simulink model "model"  (R2020a)
settings: Solver=ode4  StartTime=0.0  StopTime=simtime  FixedStep=0.001  RelTol=1e-3
values from neighbouring files (symbols this model uses):
  desired_energy = M1*g*(H+r1) + M2*g*(H+k0+r2)    (= 228.34)    [init.m]
  desired_energy2 = M1*g*(H2+r1) + M2*g*(H2+k0+r2)    (= 271.46)    [init.m]
  g = 9.8    [init.m]
  H = 0.8    [init.m]
  H2 = 1.2    [init.m]
  I1 = 1    [init.m]
  I2 = 10    [init.m]
  ini_theta1 = 0    [init.m]
  ini_theta1_d = 0    [init.m]
  ini_theta2 = 0    [init.m]
  ini_theta2_d = 0    [init.m]
  ini_x1 = ini_x0+r1*sin(ini_theta1)    [init.m]
  ini_x1_d = 0    [init.m]
  ini_x2 = ini_x1+r2*sin(ini_theta2)    [init.m]
  ini_x2_d = 0    [init.m]
  ini_y1 = ini_y0+r1*cos(ini_theta1)    [init.m]
  ini_y1_d = 0    [init.m]
  ini_y2 = ini_y0+ini_w+r2*cos(ini_theta2)    [init.m]
  ini_y2_d = 0    [init.m]
  M1 = 1    [init.m]
  M2 = 10    [init.m]
  r1 = 0.5    [init.m]
  r2 = 0.4    [init.m]
  T2_change = 50    [init.m]
settings Model: Creator=fabia  LastModifiedBy=Josè

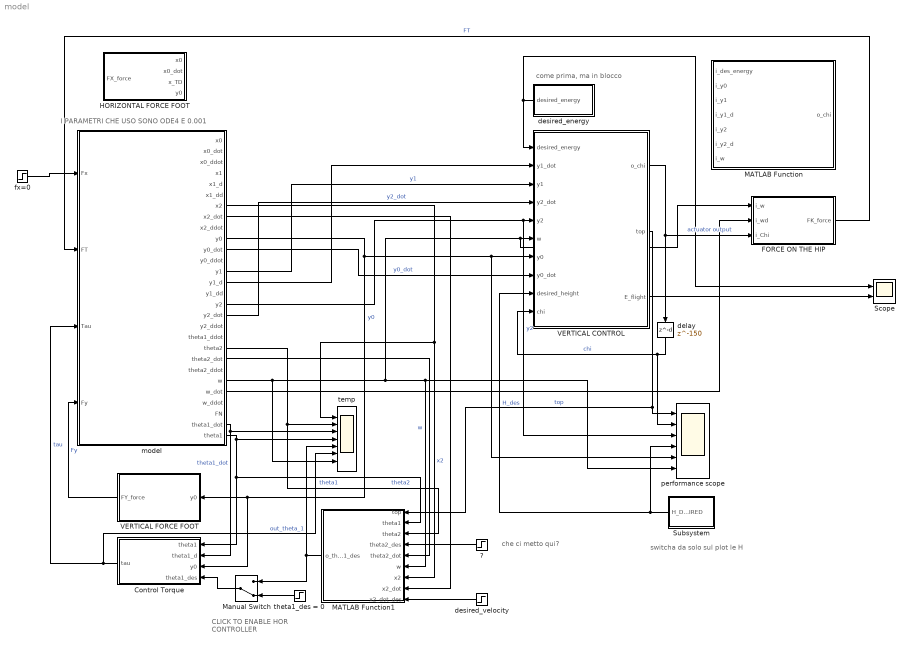
== system model ==
  note: che ci metto qui?
  note: CLICK TO ENABLE HOR CONTROLLER
  note: I PARAMETRI CHE USO SONO ODE4 E 0.001
  note: come prima, ma in blocco
  note: switcha da solo sul plot le H
  " HORIZONTAL FORCE FOOT" : MATLAB Function  TreatAsAtomicUnit=on
  " VERTICAL FORCE FOOT" : MATLAB Function  TreatAsAtomicUnit=on
  "?" : Step  Time=0  After=0  SampleTime=0
  Control Torque : MATLAB Function  TreatAsAtomicUnit=on
  FORCE ON THE HIP : MATLAB Function  TreatAsAtomicUnit=on
  MATLAB Function : MATLAB Function  TreatAsAtomicUnit=on
  MATLAB Function1 : MATLAB Function  TreatAsAtomicUnit=on
  Manual Switch : ManualSwitch  CurrentSetting=0
  Scope : Scope  NumInputPorts=2
  Subsystem : Subsystem
  VERTICAL CONTROL : MATLAB Function  TreatAsAtomicUnit=on
  delay : Delay  DelayLength=150  InitialCondition=0
  desired_energy : Subsystem
  desired_velocity : Step  Time=0  After=0.1  SampleTime=0
  fx=0 : Step  Time=0  After=0  SampleTime=0
  model : Subsystem
  performance scope : Scope  NumInputPorts=6
  temp : Scope  NumInputPorts=7
  theta1_des = 0 : Step  Time=0  After=0  SampleTime=0
  wires:
  VERTICAL CONTROL/1(o_chi) -> FORCE ON THE HIP/3(i_Chi), delay/1  "actuator output"
  fx=0/1 -> model/1(Fx)
  desired_energy/1(desired_energy) -> Scope/1, VERTICAL CONTROL/1(desired_energy)
  delay/1 -> performance scope/2, VERTICAL CONTROL/10(chi)  "chi"
  Subsystem/1(H_DESIRED) -> performance scope/4, VERTICAL CONTROL/9(desired_height)  "H_des"
  model/16(y2) -> performance scope/3, VERTICAL CONTROL/5(y2)  "y2"
  model/23(w) -> performance scope/6, MATLAB Function1/6(w), FORCE ON THE HIP/1(i_w), VERTICAL CONTROL/6(w), temp/7  "w"
  model/10(y0) -> Control Torque/3(y0), " VERTICAL FORCE FOOT"/1(y0), performance scope/5, VERTICAL CONTROL/7(y0)  "y0"
  model/11(y0_dot) -> VERTICAL CONTROL/8(y0_dot)  "y0_dot"
  model/13(y1) -> VERTICAL CONTROL/3(y1)  "y1"
  model/17(y2_dot) -> VERTICAL CONTROL/4(y2_dot)  "y2_dot"
  model/14(y1_d) -> VERTICAL CONTROL/2(y1_dot)
  " VERTICAL FORCE FOOT"/1(FY_force) -> model/4(Fy)  "Fy"
  FORCE ON THE HIP/1(FK_force) -> model/2(FT)  "FT"
  model/24(w_dot) -> FORCE ON THE HIP/2(i_wd)
  Control Torque/1(tau) -> temp/6, model/3(Tau)  "tau"
  model/28(theta1) -> MATLAB Function1/2(theta1), Control Torque/1(theta1), temp/4  "theta1"
  model/27(theta1_dot) -> Control Torque/2(theta1_d), temp/3  "theta1_dot"
  model/20(theta2) -> temp/2, MATLAB Function1/3(theta2)  "theta2"
  VERTICAL CONTROL/2(top) -> MATLAB Function1/1(top), performance scope/1  "top"
  "?"/1 -> MATLAB Function1/4(theta2_des)
  model/21(theta2_dot) -> MATLAB Function1/5(theta2_dot)
  model/7(x2) -> temp/1, MATLAB Function1/7(x2)  "x2"
  model/8(x2_dot) -> MATLAB Function1/8(x2_dot)
  desired_velocity/1 -> MATLAB Function1/9(x2_dot_des)
  MATLAB Function1/1(o_theta1_des) -> Manual Switch/1, temp/5  "out_theta_1"
  Manual Switch/1 -> Control Torque/4(theta1_des)
  theta1_des = 0/1 -> Manual Switch/2
  VERTICAL CONTROL/3(E_flight) -> Scope/2

== system model/Subsystem ==
  Add1 : Sum  Inputs=+-+
  Step1 : Step  Time=T2_change  After=H  SampleTime=0
  Step4 : Step  Time=T2_change  After=H2  SampleTime=0
  initial1 : Step  Time=0  After=H  SampleTime=0
  H_DESIRED : Outport
  wires:
  Step4/1 -> Add1/3
  Step1/1 -> Add1/2
  initial1/1 -> Add1/1
  Add1/1 -> H_DESIRED/1  "H_DESIRED"

== system model/desired_energy ==
  Add : Sum  Inputs=+-+
  Step2 : Step  Time=T2_change  After=desired_energy  SampleTime=0
  Step3 : Step  Time=T2_change  After=desired_energy2  SampleTime=0
  initial : Step  Time=0  After=desired_energy  SampleTime=0
  desired_energy : Outport
  wires:
  initial/1 -> Add/1
  Step2/1 -> Add/2
  Step3/1 -> Add/3
  Add/1 -> desired_energy/1

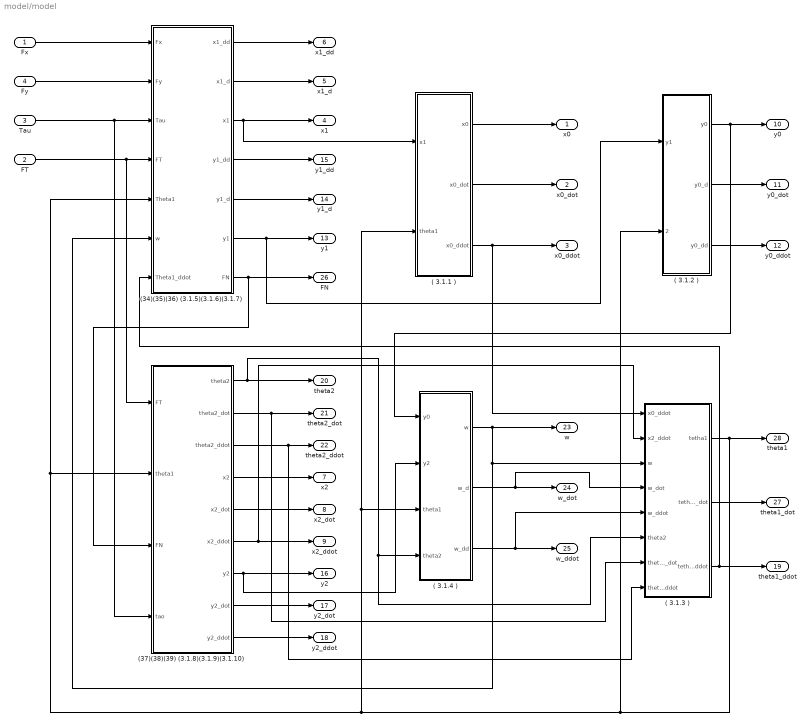
== system model/model ==
  Fx : Inport
  FT : Inport  Port=2
  Tau : Inport  Port=3
  Fy : Inport  Port=4
  "( 3.1.1 ) " : Subsystem
  ( 3.1.2 ) : Subsystem
  ( 3.1.3 ) : Subsystem
  ( 3.1.4 ) : Subsystem
  (34)(35)(36) (3.1.5)(3.1.6)(3.1.7) : Subsystem
  (37)(38)(39) (3.1.8)(3.1.9)(3.1.10) : Subsystem
  x0 : Outport
  x0_dot : Outport  Port=2
  x0_ddot : Outport  Port=3
  x1 : Outport  Port=4
  x1_d : Outport  Port=5
  x1_dd : Outport  Port=6
  x2 : Outport  Port=7
  x2_dot : Outport  Port=8
  x2_ddot : Outport  Port=9
  y0 : Outport  Port=10
  y0_dot : Outport  Port=11
  y0_ddot : Outport  Port=12
  y1 : Outport  Port=13
  y1_d : Outport  Port=14
  y1_dd : Outport  Port=15
  y2 : Outport  Port=16
  y2_dot : Outport  Port=17
  y2_ddot : Outport  Port=18
  theta1_ddot : Outport  Port=19
  theta2 : Outport  Port=20
  theta2_dot : Outport  Port=21
  theta2_ddot : Outport  Port=22
  w : Outport  Port=23
  w_dot : Outport  Port=24
  w_ddot : Outport  Port=25
  FN : Outport  Port=26
  theta1_dot : Outport  Port=27
  theta1 : Outport  Port=28
  wires:
  (34)(35)(36) (3.1.5)(3.1.6)(3.1.7)/3(x1) -> "( 3.1.1 ) "/1(x1), x1/1
  Fy/1 -> (34)(35)(36) (3.1.5)(3.1.6)(3.1.7)/2(Fy)
  Tau/1 -> (34)(35)(36) (3.1.5)(3.1.6)(3.1.7)/3(Tau), (37)(38)(39) (3.1.8)(3.1.9)(3.1.10)/4(tao)
  (34)(35)(36) (3.1.5)(3.1.6)(3.1.7)/4(y1_dd) -> y1_dd/1
  "( 3.1.1 ) "/1(x0) -> x0/1
  (34)(35)(36) (3.1.5)(3.1.6)(3.1.7)/5(y1_d) -> y1_d/1
  (34)(35)(36) (3.1.5)(3.1.6)(3.1.7)/6(y1) -> ( 3.1.2 )/1(y1), y1/1
  Fx/1 -> (34)(35)(36) (3.1.5)(3.1.6)(3.1.7)/1(Fx)
  (34)(35)(36) (3.1.5)(3.1.6)(3.1.7)/1(x1_dd) -> x1_dd/1
  "( 3.1.1 ) "/2(x0_dot) -> x0_dot/1
  (34)(35)(36) (3.1.5)(3.1.6)(3.1.7)/2(x1_d) -> x1_d/1
  (34)(35)(36) (3.1.5)(3.1.6)(3.1.7)/7(FN) -> (37)(38)(39) (3.1.8)(3.1.9)(3.1.10)/3(FN), FN/1
  "( 3.1.1 ) "/3(x0_ddot) -> x0_ddot/1, ( 3.1.3 )/1(x0_ddot)
  ( 3.1.2 )/1(y0) -> ( 3.1.4 )/1(y0), y0/1
  ( 3.1.2 )/2(y0_d) -> y0_dot/1
  ( 3.1.2 )/3(y0_dd) -> y0_ddot/1
  (37)(38)(39) (3.1.8)(3.1.9)(3.1.10)/4(x2) -> x2/1
  (37)(38)(39) (3.1.8)(3.1.9)(3.1.10)/1(theta2) -> theta2/1, ( 3.1.4 )/4(theta2), ( 3.1.3 )/6(theta2)
  (37)(38)(39) (3.1.8)(3.1.9)(3.1.10)/2(theta2_dot) -> theta2_dot/1, ( 3.1.3 )/7(theta2_dot)
  (37)(38)(39) (3.1.8)(3.1.9)(3.1.10)/3(theta2_ddot) -> theta2_ddot/1, ( 3.1.3 )/8(theta2_ddot)
  (37)(38)(39) (3.1.8)(3.1.9)(3.1.10)/5(x2_dot) -> x2_dot/1
  (37)(38)(39) (3.1.8)(3.1.9)(3.1.10)/6(x2_ddot) -> x2_ddot/1, ( 3.1.3 )/2(x2_ddot)
  (37)(38)(39) (3.1.8)(3.1.9)(3.1.10)/8(y2_dot) -> y2_dot/1
  (37)(38)(39) (3.1.8)(3.1.9)(3.1.10)/7(y2) -> y2/1, ( 3.1.4 )/2(y2)
  (37)(38)(39) (3.1.8)(3.1.9)(3.1.10)/9(y2_ddot) -> y2_ddot/1
  ( 3.1.4 )/1(w) -> ( 3.1.3 )/3(w), (34)(35)(36) (3.1.5)(3.1.6)(3.1.7)/6(w), w/1
  ( 3.1.4 )/2(w_d) -> w_dot/1, ( 3.1.3 )/4(w_dot)
  ( 3.1.4 )/3(w_dd) -> ( 3.1.3 )/5(w_ddot), w_ddot/1
  ( 3.1.3 )/1(tetha1) -> ( 3.1.2 )/2(theta1), ( 3.1.4 )/3(theta1), "( 3.1.1 ) "/2(theta1), (34)(35)(36) (3.1.5)(3.1.6)(3.1.7)/5(Theta1), (37)(38)(39) (3.1.8)(3.1.9)(3.1.10)/2(theta1), theta1/1
  ( 3.1.3 )/2(tetha1_dot) -> theta1_dot/1
  FT/1 -> (34)(35)(36) (3.1.5)(3.1.6)(3.1.7)/4(FT), (37)(38)(39) (3.1.8)(3.1.9)(3.1.10)/1(FT)
  ( 3.1.3 )/3(tetha1_ddot) -> (34)(35)(36) (3.1.5)(3.1.6)(3.1.7)/7(Theta1_ddot), theta1_ddot/1

== system model/model/( 3.1.1 )  ==
  x1 : Inport
  theta1 : Inport  Port=2
  Constant : Constant  Value=r1
  Derivative : Derivative
  Derivative1 : Derivative
  Product : Product
  Sum : Sum  Inputs=+-
  Trigonometric Function : Trigonometry
  x0 : Outport
  x0_dot : Outport  Port=2
  x0_ddot : Outport  Port=3
  wires:
  Sum/1 -> x0/1, Derivative/1
  Derivative/1 -> x0_dot/1, Derivative1/1
  theta1/1 -> Trigonometric Function/1
  Trigonometric Function/1 -> Product/1
  x1/1 -> Sum/1
  Product/1 -> Sum/2
  Derivative1/1 -> x0_ddot/1
  Constant/1 -> Product/2

== system model/model/( 3.1.2 ) ==
  y1 : Inport
  theta1 : Inport  Port=2
  Add : Sum  Inputs=+-
  Constant : Constant  Value=r1
  Derivative : Derivative
  Derivative1 : Derivative
  Product : Product
  Trigonometric Function : Trigonometry  Operator=cos
  y0 : Outport
  y0_d : Outport  Port=2
  y0_dd : Outport  Port=3
  wires:
  y1/1 -> Add/1
  theta1/1 -> Trigonometric Function/1
  Trigonometric Function/1 -> Product/2
  Add/1 -> Derivative/1, y0/1
  Derivative/1 -> y0_d/1, Derivative1/1
  Derivative1/1 -> y0_dd/1
  Product/1 -> Add/2
  Constant/1 -> Product/1

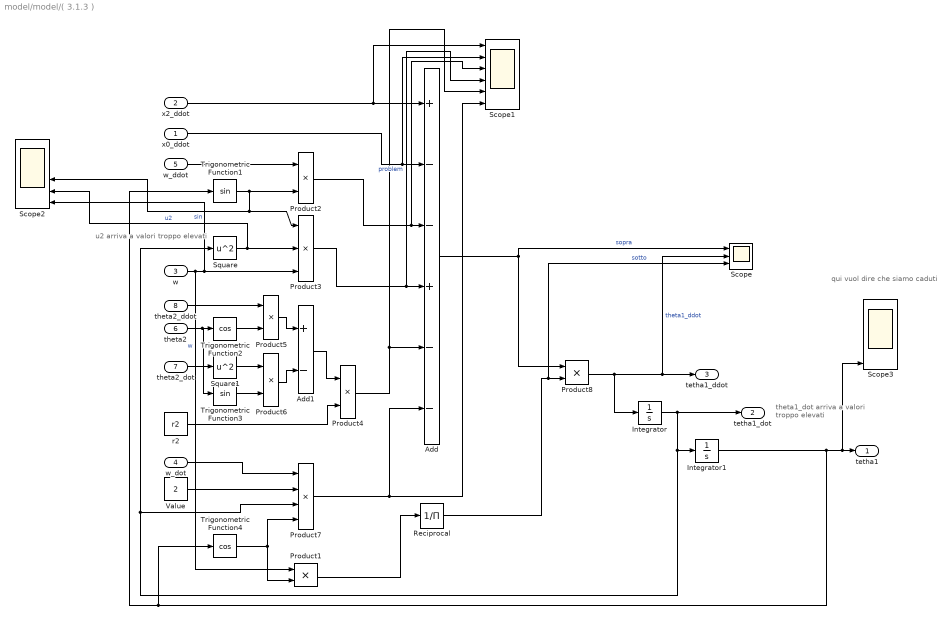
== system model/model/( 3.1.3 ) ==
  note: qui vuol dire che siamo caduti
  note: u2 arriva a valori troppo elevati
  note: theta1_dot
      | arriva a valori troppo elevati
  x0_ddot : Inport
  x2_ddot : Inport  Port=2
  w : Inport  Port=3
  w_dot : Inport  Port=4
  w_ddot : Inport  Port=5
  theta2 : Inport  Port=6
  theta2_dot : Inport  Port=7
  theta2_ddot : Inport  Port=8
  Add : Sum  Inputs=+--+--
  Add1 : Sum  Inputs=+-
  Integrator : Integrator  InitialCondition=ini_theta1_d
  Integrator1 : Integrator  InitialCondition=ini_theta1  LimitOutput=on  UpperSaturationLimit=pi/2  LowerSaturationLimit=-pi/2
  Product{1..2,4..6,8} (6 alike) : Product
  Product3 : Product  Inputs=3
  Product7 : Product  Inputs=4
  Reciprocal : Product  Inputs=/
  Scope : Scope  NumInputPorts=3
  Scope1 : Scope  NumInputPorts=6
  Scope2 : Scope  NumInputPorts=6
  Scope3 : Scope  NumInputPorts=6
  Square : Math  Operator=square  SaturateOnIntegerOverflow=on
  Square1 : Math  Operator=square  SaturateOnIntegerOverflow=on
  Trigonometric Function1 : Trigonometry
  Trigonometric Function2 : Trigonometry  Operator=cos
  Trigonometric Function3 : Trigonometry
  Trigonometric Function4 : Trigonometry  Operator=cos
  Value : Constant  Value=2
  r2 : Constant  Value=r2
  tetha1 : Outport
  tetha1_dot : Outport  Port=2
  tetha1_ddot : Outport  Port=3
  wires:
  Product8/1 -> Scope/2, tetha1_ddot/1, Integrator/1  "theta1_ddot"
  x2_ddot/1 -> Scope1/1, Add/1
  x0_ddot/1 -> Scope1/2, Add/2
  Trigonometric Function1/1 -> Product2/2, Product3/1, Scope2/4  "sin"
  w_ddot/1 -> Product2/1
  Product2/1 -> Scope1/3, Add/3
  Integrator/1 -> Square/1, Product7/3, Integrator1/1, tetha1_dot/1
  Square/1 -> Scope2/5, Product3/2  "u2"
  w/1 -> Scope2/6, Product3/3, Product1/1  "w"
  Product3/1 -> Scope1/4, Add/4  "problem"
  theta2/1 -> Trigonometric Function2/1, Trigonometric Function3/1
  Trigonometric Function2/1 -> Product5/2
  theta2_ddot/1 -> Product5/1
  Product5/1 -> Add1/1
  theta2_dot/1 -> Square1/1
  Square1/1 -> Product6/1
  Product6/1 -> Add1/2
  Trigonometric Function3/1 -> Product6/2
  r2/1 -> Product4/2
  Add1/1 -> Product4/1
  Product4/1 -> Scope1/5, Add/5
  Value/1 -> Product7/2
  w_dot/1 -> Product7/1
  Trigonometric Function4/1 -> Product1/2, Product7/4
  Product7/1 -> Scope1/6, Add/6
  Product1/1 -> Reciprocal/1
  Add/1 -> Product8/1, Scope/1  "sopra"
  Reciprocal/1 -> Scope/3, Product8/2  "sotto"
  Integrator1/1 -> Trigonometric Function4/1, Trigonometric Function1/1, Scope3/6, tetha1/1

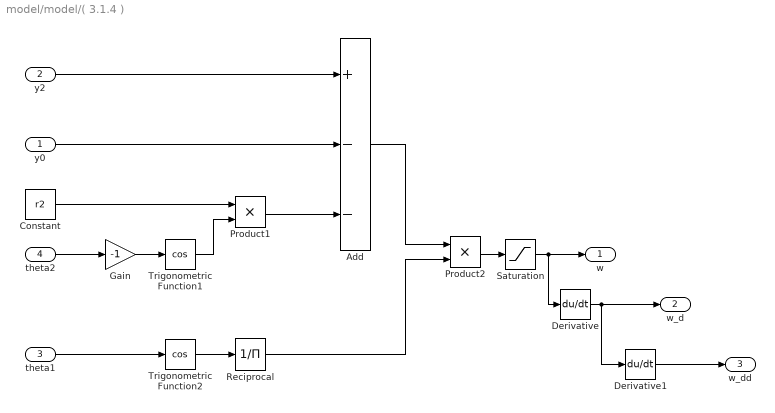
== system model/model/( 3.1.4 ) ==
  y0 : Inport
  y2 : Inport  Port=2
  theta1 : Inport  Port=3
  theta2 : Inport  Port=4
  Add : Sum  Inputs=+--
  Constant : Constant  Value=r2
  Derivative : Derivative
  Derivative1 : Derivative
  Gain : Gain  Gain=-1
  Product1 : Product
  Product2 : Product
  Reciprocal : Product  Inputs=/
  Saturation : Saturate  UpperLimit=1.6  LowerLimit=0.2
  Trigonometric Function1 : Trigonometry  Operator=cos
  Trigonometric Function2 : Trigonometry  Operator=cos
  w : Outport
  w_d : Outport  Port=2
  w_dd : Outport  Port=3
  wires:
  y2/1 -> Add/1
  theta2/1 -> Gain/1
  Gain/1 -> Trigonometric Function1/1
  Trigonometric Function1/1 -> Product1/2
  Constant/1 -> Product1/1
  Product1/1 -> Add/3
  Derivative/1 -> w_d/1, Derivative1/1
  Derivative1/1 -> w_dd/1
  y0/1 -> Add/2
  Reciprocal/1 -> Product2/2
  Add/1 -> Product2/1
  Trigonometric Function2/1 -> Reciprocal/1
  theta1/1 -> Trigonometric Function2/1
  Product2/1 -> Saturation/1
  Saturation/1 -> Derivative/1, w/1

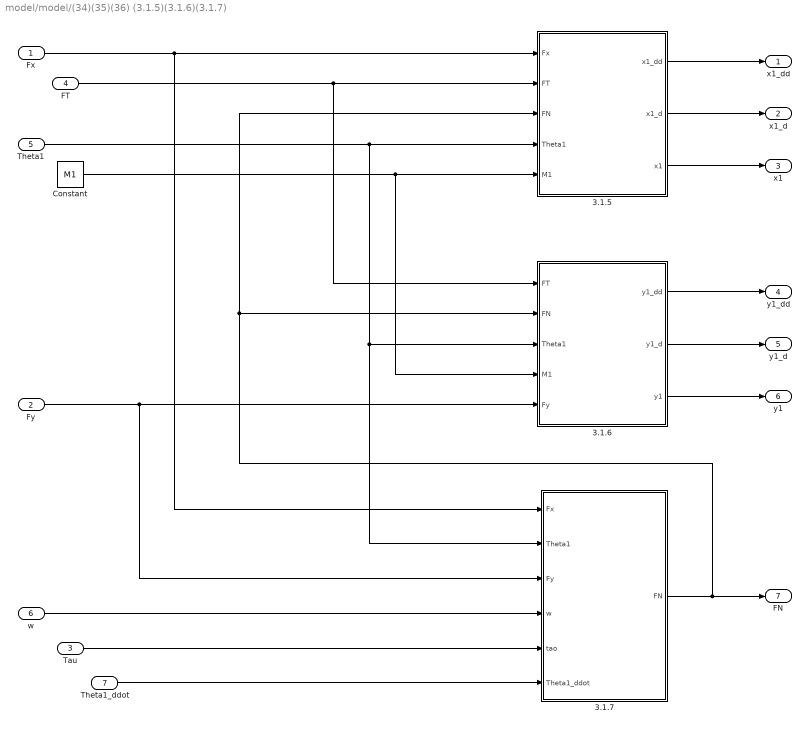
== system model/model/(34)(35)(36) (3.1.5)(3.1.6)(3.1.7) ==
  Fx : Inport
  Fy : Inport  Port=2
  Tau : Inport  Port=3
  FT : Inport  Port=4
  Theta1 : Inport  Port=5
  w : Inport  Port=6
  Theta1_ddot : Inport  Port=7
  3.1.5 : Subsystem
  3.1.6 : Subsystem
  3.1.7 : Subsystem
  Constant : Constant  Value=M1
  x1_dd : Outport
  x1_d : Outport  Port=2
  x1 : Outport  Port=3
  y1_dd : Outport  Port=4
  y1_d : Outport  Port=5
  y1 : Outport  Port=6
  FN : Outport  Port=7
  wires:
  3.1.6/2(y1_d) -> y1_d/1
  3.1.5/3(x1) -> x1/1
  3.1.5/2(x1_d) -> x1_d/1
  3.1.6/1(y1_dd) -> y1_dd/1
  Theta1/1 -> 3.1.7/2(Theta1), 3.1.6/3(Theta1), 3.1.5/4(Theta1)
  Fx/1 -> 3.1.5/1(Fx), 3.1.7/1(Fx)
  3.1.6/3(y1) -> y1/1
  3.1.7/1(FN) -> 3.1.5/3(FN), 3.1.6/2(FN), FN/1
  Tau/1 -> 3.1.7/5(tao)
  3.1.5/1(x1_dd) -> x1_dd/1
  Fy/1 -> 3.1.6/5(Fy), 3.1.7/3(Fy)
  FT/1 -> 3.1.5/2(FT), 3.1.6/1(FT)
  w/1 -> 3.1.7/4(w)
  Constant/1 -> 3.1.6/4(M1), 3.1.5/5(M1)
  Theta1_ddot/1 -> 3.1.7/6(Theta1_ddot)

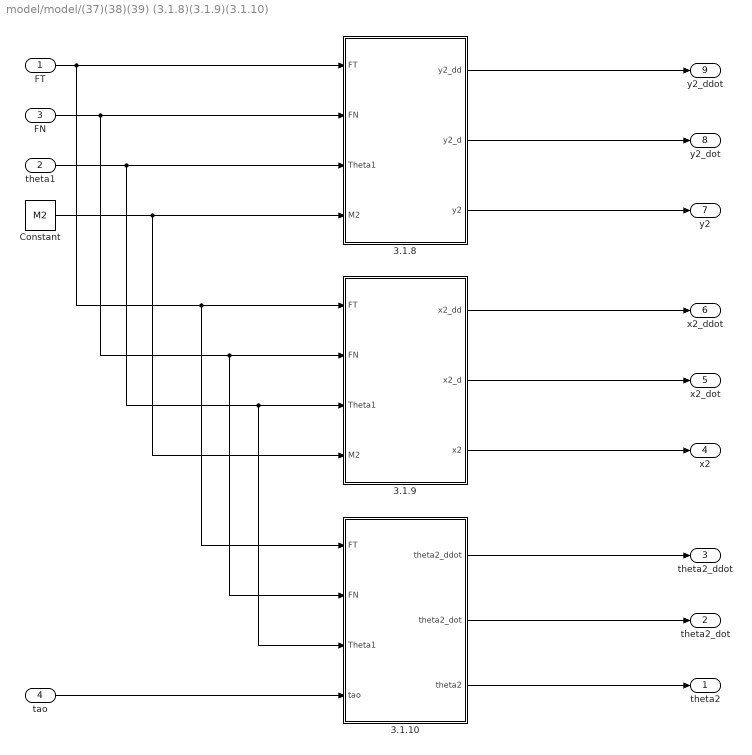
== system model/model/(37)(38)(39) (3.1.8)(3.1.9)(3.1.10) ==
  FT : Inport
  theta1 : Inport  Port=2
  FN : Inport  Port=3
  tao : Inport  Port=4
  3.1.10 : Subsystem
  3.1.8 : Subsystem
  3.1.9 : Subsystem
  Constant : Constant  Value=M2
  theta2 : Outport
  theta2_dot : Outport  Port=2
  theta2_ddot : Outport  Port=3
  x2 : Outport  Port=4
  x2_dot : Outport  Port=5
  x2_ddot : Outport  Port=6
  y2 : Outport  Port=7
  y2_dot : Outport  Port=8
  y2_ddot : Outport  Port=9
  wires:
  3.1.10/1(theta2_ddot) -> theta2_ddot/1
  3.1.10/2(theta2_dot) -> theta2_dot/1
  3.1.10/3(theta2) -> theta2/1
  3.1.8/1(y2_dd) -> y2_ddot/1
  3.1.8/2(y2_d) -> y2_dot/1
  3.1.8/3(y2) -> y2/1
  3.1.9/1(x2_dd) -> x2_ddot/1
  3.1.9/2(x2_d) -> x2_dot/1
  3.1.9/3(x2) -> x2/1
  FT/1 -> 3.1.8/1(FT), 3.1.9/1(FT), 3.1.10/1(FT)
  FN/1 -> 3.1.8/2(FN), 3.1.9/2(FN), 3.1.10/2(FN)
  theta1/1 -> 3.1.8/3(Theta1), 3.1.9/3(Theta1), 3.1.10/3(Theta1)
  Constant/1 -> 3.1.8/4(M2), 3.1.9/4(M2)
  tao/1 -> 3.1.10/4(tao)

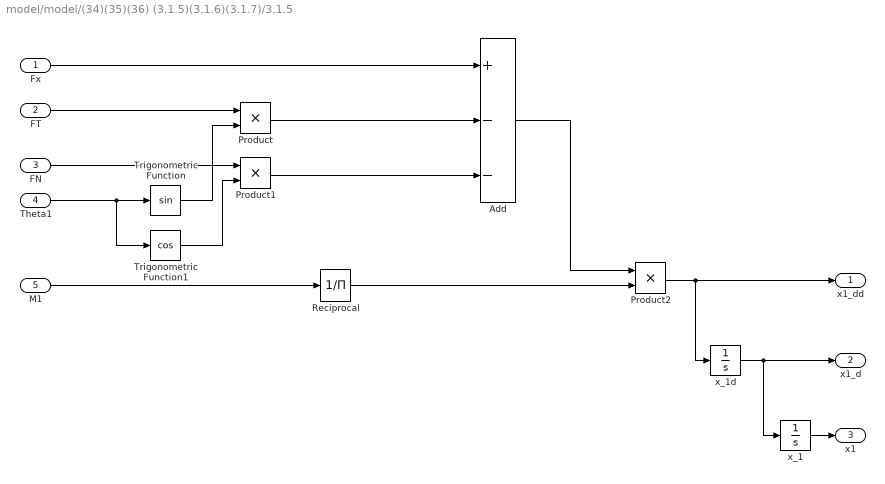
== system model/model/(34)(35)(36) (3.1.5)(3.1.6)(3.1.7)/3.1.5 ==
  Fx : Inport
  FT : Inport  Port=2
  FN : Inport  Port=3
  Theta1 : Inport  Port=4
  M1 : Inport  Port=5
  Add : Sum  Inputs=+--
  Product : Product
  Product1 : Product
  Product2 : Product
  Reciprocal : Product  Inputs=/
  Trigonometric Function : Trigonometry
  Trigonometric Function1 : Trigonometry  Operator=cos
  x_1 : Integrator  InitialCondition=ini_x1
  x_1d : Integrator  InitialCondition=ini_x1_d
  x1_dd : Outport
  x1_d : Outport  Port=2
  x1 : Outport  Port=3
  wires:
  Add/1 -> Product2/1
  FN/1 -> Product1/1
  Reciprocal/1 -> Product2/2
  Trigonometric Function1/1 -> Product1/2
  Theta1/1 -> Trigonometric Function/1, Trigonometric Function1/1
  Product1/1 -> Add/3
  Trigonometric Function/1 -> Product/2
  Product2/1 -> x_1d/1, x1_dd/1
  Product/1 -> Add/2
  FT/1 -> Product/1
  Fx/1 -> Add/1
  M1/1 -> Reciprocal/1
  x_1d/1 -> x_1/1, x1_d/1
  x_1/1 -> x1/1

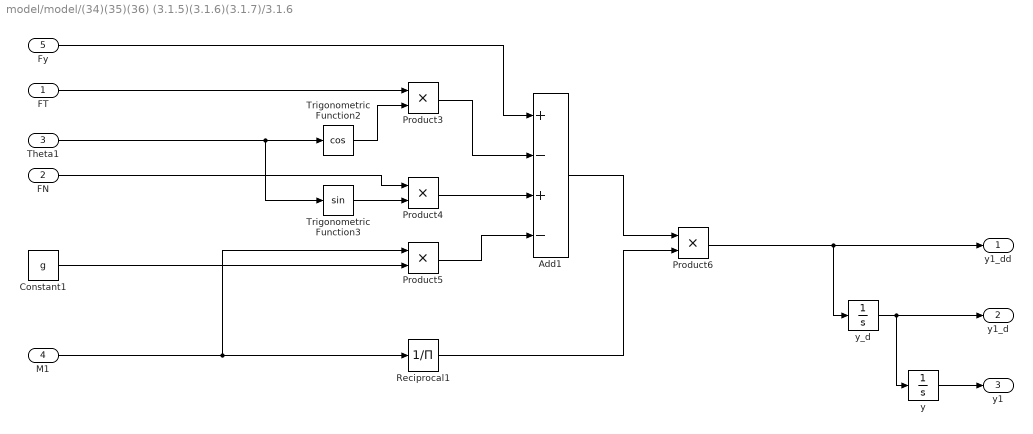
== system model/model/(34)(35)(36) (3.1.5)(3.1.6)(3.1.7)/3.1.6 ==
  FT : Inport
  FN : Inport  Port=2
  Theta1 : Inport  Port=3
  M1 : Inport  Port=4
  Fy : Inport  Port=5
  Add1 : Sum  Inputs=+-+-
  Constant1 : Constant  Value=g
  Product{3..6} (4 alike) : Product
  Reciprocal1 : Product  Inputs=/
  Trigonometric Function2 : Trigonometry  Operator=cos
  Trigonometric Function3 : Trigonometry
  y : Integrator  InitialCondition=ini_y1
  y_d : Integrator  InitialCondition=ini_y1_d
  y1_dd : Outport
  y1_d : Outport  Port=2
  y1 : Outport  Port=3
  wires:
  Product3/1 -> Add1/2
  Product4/1 -> Add1/3
  Theta1/1 -> Trigonometric Function2/1, Trigonometric Function3/1
  M1/1 -> Product5/1, Reciprocal1/1
  Trigonometric Function3/1 -> Product4/2
  Trigonometric Function2/1 -> Product3/2
  Reciprocal1/1 -> Product6/2
  Product5/1 -> Add1/4
  Add1/1 -> Product6/1
  Fy/1 -> Add1/1
  Constant1/1 -> Product5/2
  FT/1 -> Product3/1
  FN/1 -> Product4/1
  Product6/1 -> y_d/1, y1_dd/1
  y_d/1 -> y/1, y1_d/1
  y/1 -> y1/1

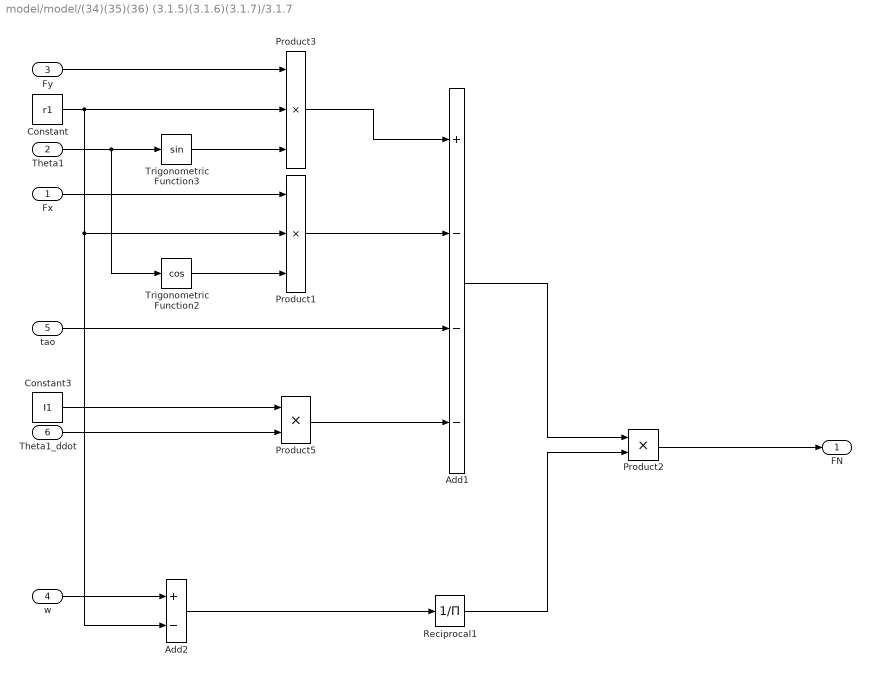
== system model/model/(34)(35)(36) (3.1.5)(3.1.6)(3.1.7)/3.1.7 ==
  Fx : Inport
  Theta1 : Inport  Port=2
  Fy : Inport  Port=3
  w : Inport  Port=4
  tao : Inport  Port=5
  Theta1_ddot : Inport  Port=6
  Add1 : Sum  Inputs=+---
  Add2 : Sum  Inputs=+-
  Constant : Constant  Value=r1
  Constant3 : Constant  Value=I1
  Product1 : Product  Inputs=3
  Product2 : Product
  Product3 : Product  Inputs=3
  Product5 : Product
  Reciprocal1 : Product  Inputs=/
  Trigonometric Function2 : Trigonometry  Operator=cos
  Trigonometric Function3 : Trigonometry
  FN : Outport
  wires:
  Product2/1 -> FN/1
  Constant/1 -> Product3/2, Product1/2, Add2/2
  Fy/1 -> Product3/1
  Theta1/1 -> Trigonometric Function3/1, Trigonometric Function2/1
  Trigonometric Function3/1 -> Product3/3
  Product3/1 -> Add1/1
  Fx/1 -> Product1/1
  Trigonometric Function2/1 -> Product1/3
  Product1/1 -> Add1/2
  tao/1 -> Add1/3
  w/1 -> Add2/1
  Add2/1 -> Reciprocal1/1
  Constant3/1 -> Product5/1
  Product5/1 -> Add1/4
  Reciprocal1/1 -> Product2/2
  Add1/1 -> Product2/1
  Theta1_ddot/1 -> Product5/2

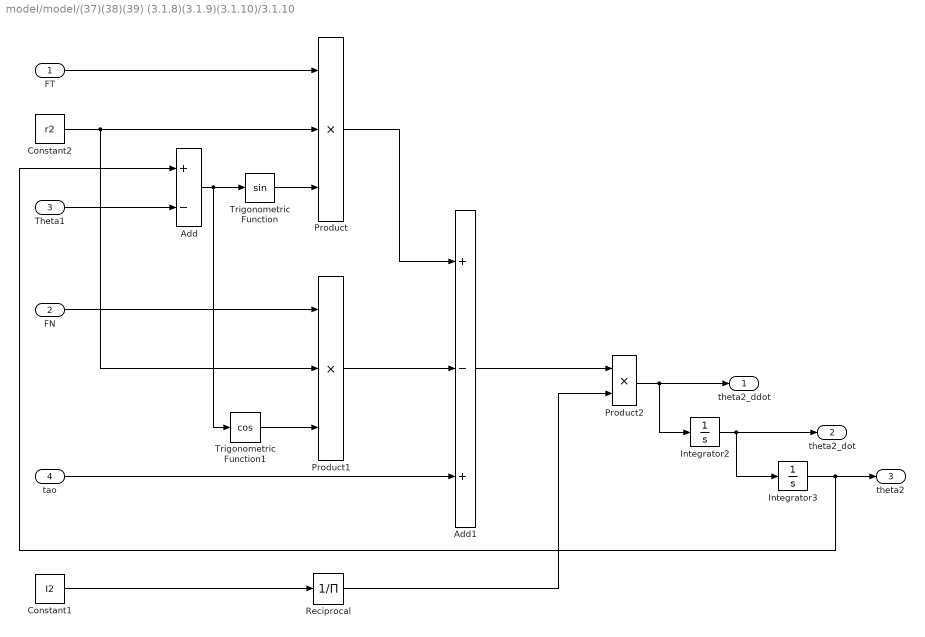
== system model/model/(37)(38)(39) (3.1.8)(3.1.9)(3.1.10)/3.1.10 ==
  FT : Inport
  FN : Inport  Port=2
  Theta1 : Inport  Port=3
  tao : Inport  Port=4
  Add : Sum  Inputs=+-
  Add1 : Sum  Inputs=+-+
  Constant1 : Constant  Value=I2
  Constant2 : Constant  Value=r2
  Integrator2 : Integrator  InitialCondition=ini_theta2_d
  Integrator3 : Integrator  InitialCondition=ini_theta2  LimitOutput=on  UpperSaturationLimit=pi/2  LowerSaturationLimit=-pi/2
  Product : Product  Inputs=3
  Product1 : Product  Inputs=3
  Product2 : Product
  Reciprocal : Product  Inputs=/
  Trigonometric Function : Trigonometry
  Trigonometric Function1 : Trigonometry  Operator=cos
  theta2_ddot : Outport
  theta2_dot : Outport  Port=2
  theta2 : Outport  Port=3
  wires:
  Product2/1 -> Integrator2/1, theta2_ddot/1
  Integrator2/1 -> Integrator3/1, theta2_dot/1
  Integrator3/1 -> Add/1, theta2/1
  Theta1/1 -> Add/2
  Add/1 -> Trigonometric Function1/1, Trigonometric Function/1
  Trigonometric Function/1 -> Product/3
  Constant2/1 -> Product/2, Product1/2
  FT/1 -> Product/1
  FN/1 -> Product1/1
  Trigonometric Function1/1 -> Product1/3
  Product1/1 -> Add1/2
  Product/1 -> Add1/1
  tao/1 -> Add1/3
  Constant1/1 -> Reciprocal/1
  Reciprocal/1 -> Product2/2
  Add1/1 -> Product2/1

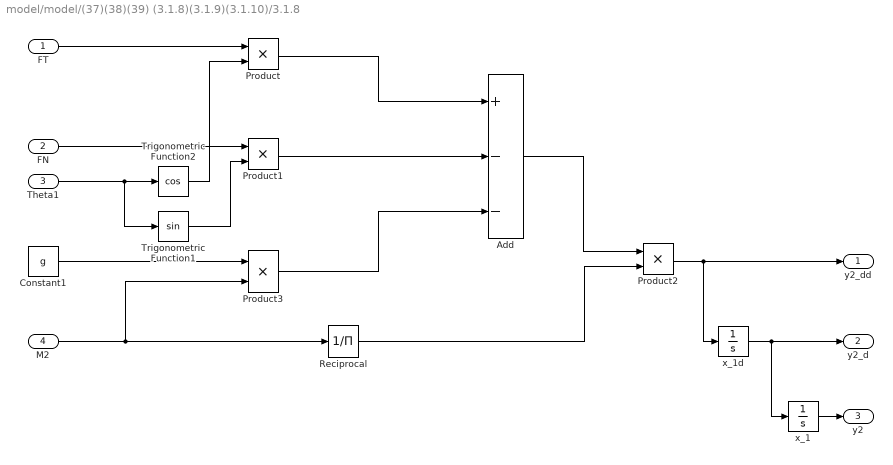
== system model/model/(37)(38)(39) (3.1.8)(3.1.9)(3.1.10)/3.1.8 ==
  FT : Inport
  FN : Inport  Port=2
  Theta1 : Inport  Port=3
  M2 : Inport  Port=4
  Add : Sum  Inputs=+--
  Constant1 : Constant  Value=g
  Product{,1..3} (4 alike) : Product
  Reciprocal : Product  Inputs=/
  Trigonometric Function1 : Trigonometry
  Trigonometric Function2 : Trigonometry  Operator=cos
  x_1 : Integrator  InitialCondition=ini_y2
  x_1d : Integrator  InitialCondition=ini_y2_d
  y2_dd : Outport
  y2_d : Outport  Port=2
  y2 : Outport  Port=3
  wires:
  Add/1 -> Product2/1
  FN/1 -> Product1/1
  Reciprocal/1 -> Product2/2
  Trigonometric Function1/1 -> Product1/2
  Theta1/1 -> Trigonometric Function2/1, Trigonometric Function1/1
  Product2/1 -> x_1d/1, y2_dd/1
  FT/1 -> Product/1
  M2/1 -> Reciprocal/1, Product3/2
  x_1d/1 -> x_1/1, y2_d/1
  x_1/1 -> y2/1
  Trigonometric Function2/1 -> Product/2
  Product/1 -> Add/1
  Product1/1 -> Add/2
  Constant1/1 -> Product3/1
  Product3/1 -> Add/3

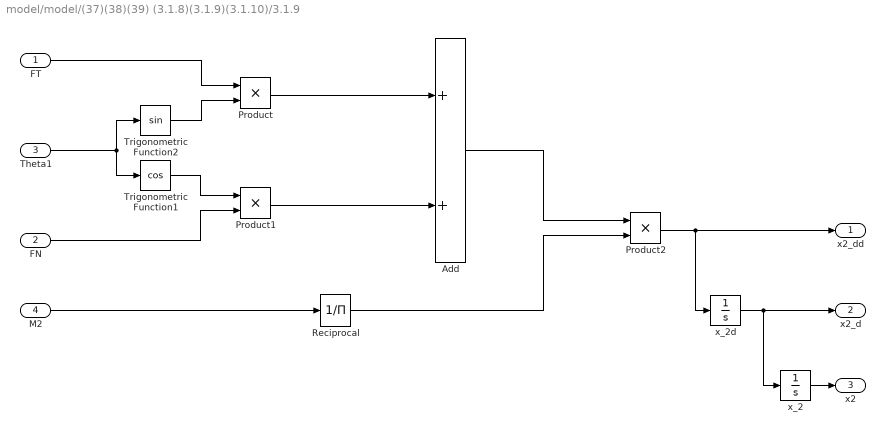
== system model/model/(37)(38)(39) (3.1.8)(3.1.9)(3.1.10)/3.1.9 ==
  FT : Inport
  FN : Inport  Port=2
  Theta1 : Inport  Port=3
  M2 : Inport  Port=4
  Add : Sum
  Product : Product
  Product1 : Product
  Product2 : Product
  Reciprocal : Product  Inputs=/
  Trigonometric Function1 : Trigonometry  Operator=cos
  Trigonometric Function2 : Trigonometry
  x_2 : Integrator  InitialCondition=ini_x2
  x_2d : Integrator  InitialCondition=ini_x2_d
  x2_dd : Outport
  x2_d : Outport  Port=2
  x2 : Outport  Port=3
  wires:
  Add/1 -> Product2/1
  Reciprocal/1 -> Product2/2
  Theta1/1 -> Trigonometric Function2/1, Trigonometric Function1/1
  Product2/1 -> x_2d/1, x2_dd/1
  FT/1 -> Product/1
  M2/1 -> Reciprocal/1
  x_2d/1 -> x_2/1, x2_d/1
  x_2/1 -> x2/1
  Trigonometric Function2/1 -> Product/2
  Product/1 -> Add/1
  Product1/1 -> Add/2
  FN/1 -> Product1/2
  Trigonometric Function1/1 -> Product1/1

== matlab function model/ VERTICAL FORCE FOOT ==
  data: y0 input; FY_force output
function FY_force = Fy(y0)

KG=10^4; % [Nt/m]
BG=75; % [Nt-s/m]

FY_force = 0;

if y0<0 
    FY_force = -KG*y0-BG*y0;
end

== matlab function model/VERTICAL CONTROL ==
  data: desired_energy input; y1_dot input; y1 input; y2_dot input; y2 input; w input; y0 input; o_chi output; y0_dot input; desired_height input; chi input; top output; E_flight output
function [o_chi,top,E_flight]  = Vertical_control(desired_energy,y1_dot,y1,y2_dot,y2,w,y0, y0_dot,desired_height,chi)

chi_min=0.00;
chi_max=0.2;

M1=1; % Leg mass [kg]
M2=10; % Body mass [kg]

k0=1; % [m]
KL=10^3; % [Nt/m]

KG=10^4; % [Nt/m]
g=9.8;

E_flight=(M2/(M1+M2))*...
    (M1*g*y1+...
    M2*g*y2+...
    0.5*M1*y1_dot^2+...
    0.5*M2*y2_dot^2+...
    0.5*(KL*(k0-w+chi)^2)+...
    0.5*KG*y0^2);

Delta_EH=desired_energy-E_flight;

Delta_chi=-(chi-w+k0)+sqrt((chi-w+k0)^2+((2*abs(Delta_EH))/KL));

if Delta_EH >= 0
    o_chi=chi+Delta_chi;
else
    o_chi=chi-Delta_chi;
end

%
if o_chi<chi_min
    o_chi=chi_min;
end
if o_chi>chi_max
    o_chi=chi_max;
end

top = 0;

% this is used to understand TOP configuration, so when the hopper is at
% the maximum height
if ( y0 > 0.1 )&& (y2_dot >=-0.0095 && y2_dot<=0.0095)
    % here i understand when  it's in top state
    top = 1;
end





































% ----------------------------michele-----------------------------------

% % INIT VARIABLE, IF USED BELOW
% jumping_error =0;
%
% M1=1; % Leg mass [kg]
% M2=10; % Body mass [kg]
%
% k0=1; % [m]
% KL=10^3; % [Nt/m]
%
% KG=10^4; % [Nt/m]
% g=9.8;
%
%
% current_jumping_height = 0;
% chi_min=0.0;
% chi_max=0.2;
%
%
% E_flight=(M2/(M1+M2))*...
%     (M1*g*y1+...
%     M2*g*y2+...
%     0.5*M1*y1_dot^2+...
%     0.5*M2*y2_dot^2+...
%     0.5*(KL*(k0-w+chi)^2)+...
%     0.5*KG*y0^2);
%
% Delta_EH= abs(desired_energy-E_flight);
%
% Delta_chi=-(chi-w+k0)+sqrt((chi-w+k0)^2+((2*(Delta_EH))/KL));
%
% if Delta_EH >= 0
%     o_chi=chi+Delta_chi;
% else
%     o_chi=chi-Delta_chi;
% end
%
% if o_chi<chi_min
%     o_chi=chi_min;
% end
% if o_chi>chi_max
%     o_chi=chi_max;
% end
%
% %%
% % this is used to understand TOP configuration, so when the hopper is at
% % the maximum height
% if ( o_chi==0 )&& (y0_dot>=-0.0085 && y0_dot<=0.0085)
%     % here i understand when  it's in top state
%     top = 1;
%     % also i know its current height
%     current_jumping_height = y0;
%     % here i get the jumping error
%     jumping_error = (desired_height - current_jumping_height);
%
%
% else top = 0;
% end
%
% % SINCE IT SEAMS THAT IF YOU POT H=0.4 IT JUMPS AT 0.35
%
% % HERE THE IDEA IS TO AUGMENT CHI BY THAT ERROR IN HEIGHT IT HAS
% % IN FACT IF YOU PUT o_chi=  o_chi*(1+(H=0.4-0.35)) IT REACHES THE
% % CORRECT HEIGHT
% % if jumping_error > 0
% %     o_chi=  o_chi*(1+jumping_error);
% % end
end

== matlab function model/FORCE ON THE HIP ==
  data: i_w input; FK_force output; i_wd input; i_Chi input
function FK_force  = FK(i_w,i_wd,i_Chi)

k0=1; % [m]
KL=10^3; % [Nt/m]

KL2=10^5; % [Nt/m]
BL2=125; % [Nt-s/m]

condition = (k0-i_w+i_Chi);

FK_force=KL2*condition-(BL2*i_wd);


if condition>0
    FK_force = KL*condition;
end

    
end

== matlab function model/Control Torque ==
  data: theta1 input; theta1_d input; y0 input; tau output; theta1_des input
function tau = fcn(theta1,theta1_d,y0, theta1_des)

if y0<=0
    Kp=1800; %[Nt-m/rad]
    Kv=200; %[Nt-m-s/rad]
else
    Kp=1200; %[Nt-m/rad]
    Kv=60; %[Nt-m-s/rad]
end
tau=Kp*(theta1-theta1_des)+Kv*(theta1_d);

== matlab function model/MATLAB Function ==
  data: i_des_energy input; o_chi output; i_y0 input; i_y1 input; i_y1_d input; i_y2 input; i_y2_d input; i_w input
function o_chi = Fabian_Vertical_control(i_des_energy,i_y0,i_y1,i_y1_d,i_y2,i_y2_d,i_w)

chi_min=0.00;
chi_max=0.25;

M1=1; % Leg mass [kg]
M2=10; % Body mass [kg]

k0=1; % [m]
KL=10^3; % [Nt/m]

KG=10^4; % [Nt/m]
g=9.8;

E_flight=(M2/(M1+M2))*...
    (M1*g*i_y1+...
    M2*g*i_y2+...
    0.5*M1*i_y1_d^2+...
    0.5*M2*i_y2_d^2+...
    0.5*(KL*(k0-i_w+chi_min)^2)+...
    0.5*KG*i_y0^2);

Delta_EH=i_des_energy-E_flight;

Delta_chi=-(chi_min-i_w+k0)+sqrt((chi_min-i_w+k0)^2+((2*abs(Delta_EH))/KL));

if Delta_EH >= 0
    o_chi=chi_min+Delta_chi;
else
    o_chi=chi_min-Delta_chi;
end

if o_chi<chi_min
    o_chi=chi_min;
end
if o_chi>chi_max
    o_chi=chi_max;
end

== matlab function model/ HORIZONTAL FORCE FOOT ==
  data: x0 input; FX_force output; x0_dot input; x_TD input; y0 input
function FX_force = Fx(x0,x0_dot,x_TD,y0)

KG=10^4; % [Nt/m]
BG=75; % [Nt-s/m]

FX_force = 0;

if y0<0 
    FX_force = -KG*(x0-x_TD)-BG*x0_dot;
end

== matlab function model/MATLAB Function1 ==
  data: top input; theta1 input; o_theta1_des output; theta2 input; theta2_des input; theta2_dot input; w input; x2 input; x2_dot input; x2_dot_des input
function o_theta1_des = Horizontal_control(top,theta1, theta2, theta2_des, theta2_dot, w, x2, x2_dot, x2_dot_des)

% DOBBIAMO ESSENZIALMENTE CAPIRE QUANDO ATTIVARE QUESTO
% CONTROLLORE. TOP E' UNA BOOLEANA [1,0]. vale 1 quando sei
% in una configurazione top.
% questo è il controllore di fabian
% il problema è chhe non so cosa mettere a theta2_des


% default params
M1=1; % Leg mass [kg]
M2=10; % Body mass [kg]
r1=0.5; % [m]
r2=0.4; % [m]

% choose which horizontal controller to apply (now only Foot Placement)
mode = 1;

    switch mode
        case 1

        % Method 1 : Foot Placement
        % This analysis is done in a coordinate system that translates with the hip

        % Control of x2 is accomplished by implementing a posisiton controller of
        % the form:
    %     x2d_dot_max = 1.5;
    %     K = 10;   
    %     x2_dot_des = min(K*(x2 - x2*1.1), x2d_dot_max);

        % Find Horizontal position of center of gravity
        x_cg = (1/( M1+M2))*((r1-w)*M1*sin(theta1) + r2*M2*sin(theta2));

        % Calculate linear combination of state errors to provide corrective
        % feedback
        [K1,K2,K3] = deal(0.18, 0.3, 0.4);
        % x2d_dot is rechieved as input
        x_err = K1*(x2_dot - x2_dot_des) + K2*(theta2 - theta2_des) + K3*(theta2_dot);

        % Place foot at touchdown (dunno if useful)
        %x_td = x_cg+x_err;

        % Foot placement wrt hip (dunno if useful)
        %x_td_hip = w*( r2*M2*sin(theta2) + (M1+M2)*x_err)/(r1*M1 + w*M2);

        % The corresponding leg angle to achieve
        %epsi = 10^-5;
        argumasin = (r2*M2*sin(theta2) + (M1+M2)*x_err)/(r1*M1 + w*M2);
        argumasin = max(min(argumasin,1),-1);
        
        % if top = 1 output is generated
        o_theta1_des = -asin(argumasin);
        %o_theta1_des = -asin((r2*M2*sin(i_theta2) + (M1+M2)*x_err)/(r1*M1 + i_w*M2));

        case 2 

        % Method 2 : Leg sweeping

        case 3

        % Method 3 : Servo attitude
    
    end
end
